simulink model "hw5_problem8"  (R2016a)
settings: Solver=VariableStepAuto  StartTime=-.005  StopTime=.5  RelTol=1e-3
values from neighbouring files (symbols this model uses):
  f_sw = 10e3    (= 10000)    [hw5.m]
  K_i_d = 10    [hw5.m]
  K_i_q = 10    [hw5.m]
  K_p_d = 100    [hw5.m]
  K_p_q = 100    [hw5.m]
  L = 3e-3    (= 0.003)    [hw5.m]
  R = .5    (= 0.5)    [hw5.m]
  theta_syn = w*t    (= 376.991118431)    [hw5.m]
  Vbus = 250    [hw5.m]
  w = 2*pi*60    (= 376.991118431)    [hw5.m]
libraries: dspsigops x4
settings Model: Creator=Seth Barger  LastModifiedBy=Seth Barger
settings DataIOCC: SaveOutput=off

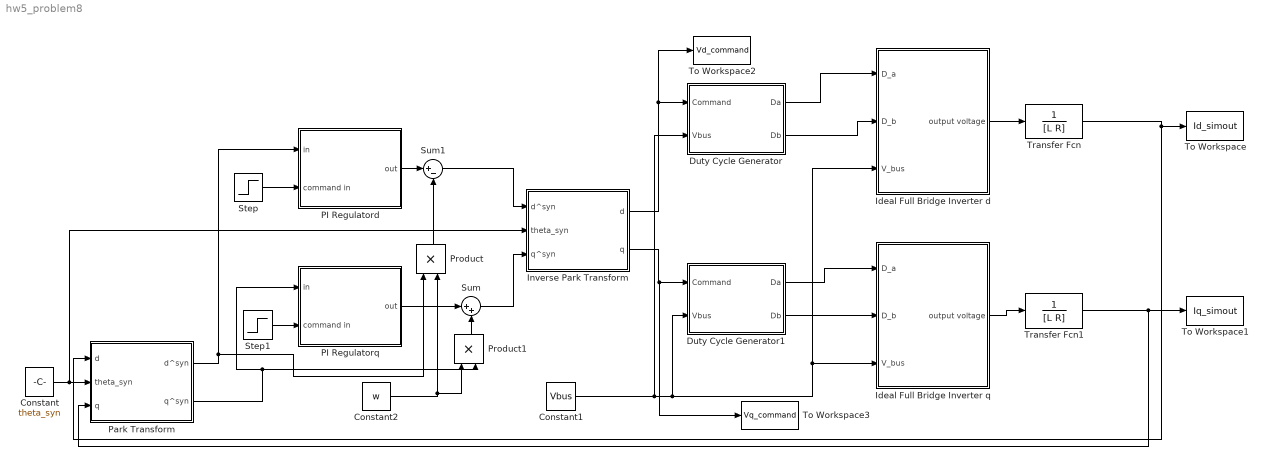
== system hw5_problem8 ==
  Constant : Constant  Value=theta_syn
  Constant1 : Constant  Value=Vbus
  Constant2 : Constant  Value=w
  Duty Cycle Generator : Subsystem
  Duty Cycle Generator1 : Subsystem
  "Ideal Full Bridge Inverter d " : Subsystem
  Ideal Full Bridge Inverter q : Subsystem
  Inverse Park Transform : Subsystem
  PI Regulatord : Subsystem
  PI Regulatorq : Subsystem
  Park Transform : Subsystem
  Product : Product
  Product1 : Product
  Step : Step  Time=0  After=20  SampleTime=0
  Step1 : Step  Time=0  After=-20  SampleTime=0
  Sum : Sum  Inputs=|++
  Sum1 : Sum  Inputs=|+-
  To Workspace : ToWorkspace  VariableName=Id_simout  SampleTime=-1
  To Workspace1 : ToWorkspace  VariableName=Iq_simout  SampleTime=-1
  To Workspace2 : ToWorkspace  VariableName=Vd_command  SampleTime=-1
  To Workspace3 : ToWorkspace  VariableName=Vq_command  SampleTime=-1
  Transfer Fcn : TransferFcn  Denominator=[L R]
  Transfer Fcn1 : TransferFcn  Denominator=[L R]
  wires:
  Constant/1 -> Inverse Park Transform/2(theta_syn), Park Transform/2(theta_syn)
  Park Transform/2(q^syn) -> Product1/2, PI Regulatorq/1(in)
  Park Transform/1(d^syn) -> Product/1, PI Regulatord/1(in)
  Constant1/1 -> Duty Cycle Generator/2(Vbus), Duty Cycle Generator1/2(Vbus), "Ideal Full Bridge Inverter d "/3(V_bus), Ideal Full Bridge Inverter q/3(V_bus)
  "Ideal Full Bridge Inverter d "/1(output voltage) -> Transfer Fcn/1
  Ideal Full Bridge Inverter q/1(output voltage) -> Transfer Fcn1/1
  Transfer Fcn1/1 -> To Workspace1/1, Park Transform/3(q)
  Transfer Fcn/1 -> To Workspace/1, Park Transform/1(d)
  Constant2/1 -> Product1/1, Product/2
  Product1/1 -> Sum/2
  PI Regulatorq/1(out) -> Sum/1
  Sum/1 -> Inverse Park Transform/3(q^syn)
  PI Regulatord/1(out) -> Sum1/1
  Product/1 -> Sum1/2
  Sum1/1 -> Inverse Park Transform/1(d^syn)
  Duty Cycle Generator/1(Da) -> "Ideal Full Bridge Inverter d "/1(D_a)
  Duty Cycle Generator/2(Db) -> "Ideal Full Bridge Inverter d "/2(D_b)
  Inverse Park Transform/1(d) -> To Workspace2/1, Duty Cycle Generator/1(Command)
  Duty Cycle Generator1/1(Da) -> Ideal Full Bridge Inverter q/1(D_a)
  Inverse Park Transform/2(q) -> To Workspace3/1, Duty Cycle Generator1/1(Command)
  Duty Cycle Generator1/2(Db) -> Ideal Full Bridge Inverter q/2(D_b)
  Step/1 -> PI Regulatord/2(command in)
  Step1/1 -> PI Regulatorq/2(command in)

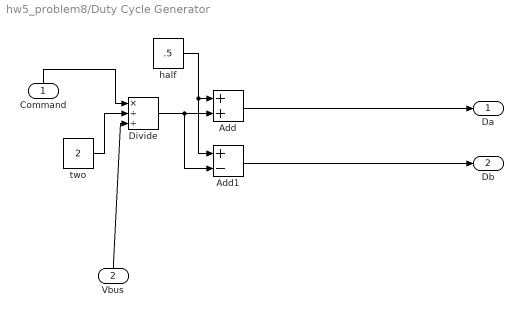
== system hw5_problem8/Duty Cycle Generator ==
  Command : Inport
  Vbus : Inport  Port=2
  Add : Sum
  Add1 : Sum  Inputs=+-
  Divide : Product  Inputs=*//
  half : Constant  Value=.5
  two : Constant  Value=2
  Da : Outport
  Db : Outport  Port=2
  wires:
  two/1 -> Divide/2
  Add/1 -> Da/1
  Command/1 -> Divide/1
  Vbus/1 -> Divide/3
  Divide/1 -> Add1/2, Add/2
  half/1 -> Add1/1, Add/1
  Add1/1 -> Db/1

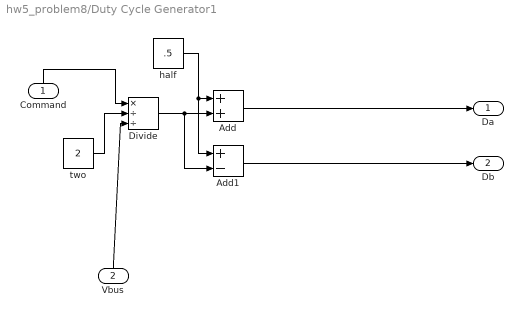
== system hw5_problem8/Duty Cycle Generator1 ==
  Command : Inport
  Vbus : Inport  Port=2
  Add : Sum
  Add1 : Sum  Inputs=+-
  Divide : Product  Inputs=*//
  half : Constant  Value=.5
  two : Constant  Value=2
  Da : Outport
  Db : Outport  Port=2
  wires:
  two/1 -> Divide/2
  Add/1 -> Da/1
  Command/1 -> Divide/1
  Vbus/1 -> Divide/3
  Divide/1 -> Add1/2, Add/2
  half/1 -> Add1/1, Add/1
  Add1/1 -> Db/1

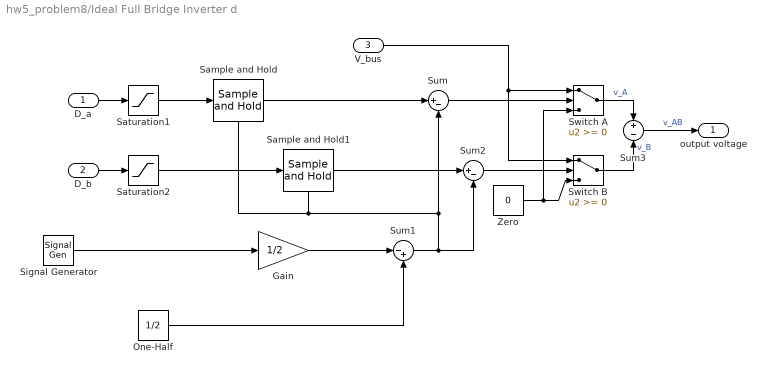
== system hw5_problem8/Ideal Full Bridge Inverter d  ==
  D_a : Inport
  D_b : Inport  Port=2
  V_bus : Inport  Port=3
  Gain : Gain  Gain=1/2  SaturateOnIntegerOverflow=on  OutDataTypeStr=Inherit: Same as input  ParamDataTypeStr=Inherit: Same as input
  One-Half : Constant  Value=1/2
  Sample and Hold : dspsigops/Sample and Hold  trig=Falling edge  initCond=0  latchinput=off
  Sample and Hold1 : dspsigops/Sample and Hold  trig=Falling edge  initCond=0  latchinput=off
  Saturation1 : Saturate  UpperLimit=1  LowerLimit=0
  Saturation2 : Saturate  UpperLimit=1  LowerLimit=0
  Signal Generator : SignalGenerator  WaveForm=sawtooth  Frequency=f_sw
  Sum : Sum  Inputs=|+-  SaturateOnIntegerOverflow=on
  Sum1 : Sum  Inputs=|-+  SaturateOnIntegerOverflow=on
  Sum2 : Sum  Inputs=|+-  SaturateOnIntegerOverflow=on
  Sum3 : Sum  Inputs=+-  SaturateOnIntegerOverflow=on
  Switch A : Switch  SaturateOnIntegerOverflow=on
  Switch B : Switch  SaturateOnIntegerOverflow=on
  Zero : Constant  Value=0
  output voltage : Outport
  wires:
  Sum/1 -> Switch A/2
  Zero/1 -> Switch A/3, Switch B/3
  Signal Generator/1 -> Gain/1
  Gain/1 -> Sum1/1
  One-Half/1 -> Sum1/2
  Sum2/1 -> Switch B/2
  Switch A/1 -> Sum3/1  "v_A"
  Switch B/1 -> Sum3/2  "v_B"
  Sum3/1 -> output voltage/1  "v_AB"
  Sum1/1 -> Sum2/2, Sample and Hold/Trigger, Sample and Hold1/Trigger, Sum/2
  V_bus/1 -> Switch A/1, Switch B/1
  D_a/1 -> Saturation1/1
  Sample and Hold/1 -> Sum/1
  D_b/1 -> Saturation2/1
  Sample and Hold1/1 -> Sum2/1
  Saturation1/1 -> Sample and Hold/1
  Saturation2/1 -> Sample and Hold1/1

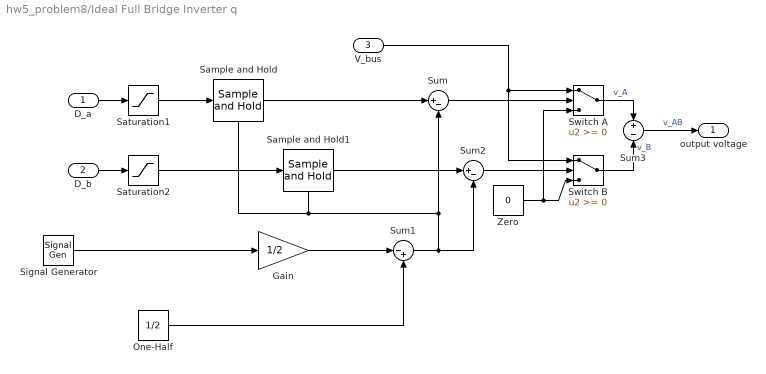
== system hw5_problem8/Ideal Full Bridge Inverter q ==
  D_a : Inport
  D_b : Inport  Port=2
  V_bus : Inport  Port=3
  Gain : Gain  Gain=1/2  SaturateOnIntegerOverflow=on  OutDataTypeStr=Inherit: Same as input  ParamDataTypeStr=Inherit: Same as input
  One-Half : Constant  Value=1/2
  Sample and Hold : dspsigops/Sample and Hold  trig=Falling edge  initCond=0  latchinput=off
  Sample and Hold1 : dspsigops/Sample and Hold  trig=Falling edge  initCond=0  latchinput=off
  Saturation1 : Saturate  UpperLimit=1  LowerLimit=0
  Saturation2 : Saturate  UpperLimit=1  LowerLimit=0
  Signal Generator : SignalGenerator  WaveForm=sawtooth  Frequency=f_sw
  Sum : Sum  Inputs=|+-  SaturateOnIntegerOverflow=on
  Sum1 : Sum  Inputs=|-+  SaturateOnIntegerOverflow=on
  Sum2 : Sum  Inputs=|+-  SaturateOnIntegerOverflow=on
  Sum3 : Sum  Inputs=+-  SaturateOnIntegerOverflow=on
  Switch A : Switch  SaturateOnIntegerOverflow=on
  Switch B : Switch  SaturateOnIntegerOverflow=on
  Zero : Constant  Value=0
  output voltage : Outport
  wires:
  Sum/1 -> Switch A/2
  Zero/1 -> Switch A/3, Switch B/3
  Signal Generator/1 -> Gain/1
  Gain/1 -> Sum1/1
  One-Half/1 -> Sum1/2
  Sum2/1 -> Switch B/2
  Switch A/1 -> Sum3/1  "v_A"
  Switch B/1 -> Sum3/2  "v_B"
  Sum3/1 -> output voltage/1  "v_AB"
  Sum1/1 -> Sum2/2, Sample and Hold/Trigger, Sample and Hold1/Trigger, Sum/2
  V_bus/1 -> Switch A/1, Switch B/1
  D_a/1 -> Saturation1/1
  Sample and Hold/1 -> Sum/1
  D_b/1 -> Saturation2/1
  Sample and Hold1/1 -> Sum2/1
  Saturation1/1 -> Sample and Hold/1
  Saturation2/1 -> Sample and Hold1/1

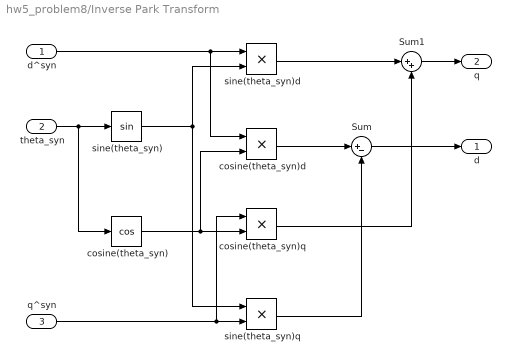
== system hw5_problem8/Inverse Park Transform ==
  d^syn : Inport
  theta_syn : Inport  Port=2
  q^syn : Inport  Port=3
  Sum : Sum  Inputs=|+-
  Sum1 : Sum  Inputs=|++
  cosine(theta_syn) : Trigonometry  Operator=cos
  cosine(theta_syn)d : Product
  cosine(theta_syn)q : Product
  sine(theta_syn) : Trigonometry
  sine(theta_syn)d : Product
  sine(theta_syn)q : Product
  d : Outport
  q : Outport  Port=2
  wires:
  Sum1/1 -> q/1
  cosine(theta_syn)q/1 -> Sum1/2
  cosine(theta_syn)d/1 -> Sum/1
  q^syn/1 -> cosine(theta_syn)q/1, sine(theta_syn)q/2
  sine(theta_syn)q/1 -> Sum/2
  cosine(theta_syn)/1 -> cosine(theta_syn)q/2, cosine(theta_syn)d/2
  Sum/1 -> d/1
  sine(theta_syn)d/1 -> Sum1/1
  theta_syn/1 -> cosine(theta_syn)/1, sine(theta_syn)/1
  d^syn/1 -> cosine(theta_syn)d/1, sine(theta_syn)d/1
  sine(theta_syn)/1 -> sine(theta_syn)q/1, sine(theta_syn)d/2

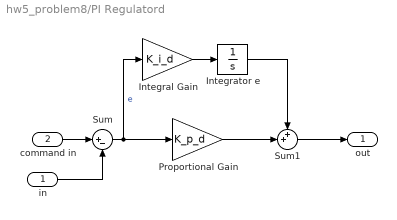
== system hw5_problem8/PI Regulatord ==
  in : Inport
  command in : Inport  Port=2
  Integral Gain : Gain  Gain=K_i_d  SaturateOnIntegerOverflow=on  OutDataTypeStr=Inherit: Same as input  ParamDataTypeStr=Inherit: Same as input
  Integrator e : Integrator
  Proportional Gain : Gain  Gain=K_p_d  SaturateOnIntegerOverflow=on  OutDataTypeStr=Inherit: Same as input  ParamDataTypeStr=Inherit: Same as input
  Sum : Sum  Inputs=|+-  SaturateOnIntegerOverflow=on
  Sum1 : Sum  Inputs=++|  SaturateOnIntegerOverflow=on
  out : Outport
  wires:
  Sum/1 -> Integral Gain/1, Proportional Gain/1  "e"
  command in/1 -> Sum/1
  in/1 -> Sum/2
  Proportional Gain/1 -> Sum1/2
  Sum1/1 -> out/1
  Integral Gain/1 -> Integrator e/1
  Integrator e/1 -> Sum1/1

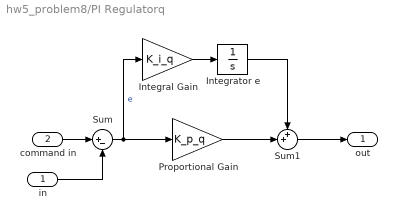
== system hw5_problem8/PI Regulatorq ==
  in : Inport
  command in : Inport  Port=2
  Integral Gain : Gain  Gain=K_i_q  SaturateOnIntegerOverflow=on  OutDataTypeStr=Inherit: Same as input  ParamDataTypeStr=Inherit: Same as input
  Integrator e : Integrator
  Proportional Gain : Gain  Gain=K_p_q  SaturateOnIntegerOverflow=on  OutDataTypeStr=Inherit: Same as input  ParamDataTypeStr=Inherit: Same as input
  Sum : Sum  Inputs=|+-  SaturateOnIntegerOverflow=on
  Sum1 : Sum  Inputs=++|  SaturateOnIntegerOverflow=on
  out : Outport
  wires:
  Sum/1 -> Integral Gain/1, Proportional Gain/1  "e"
  command in/1 -> Sum/1
  in/1 -> Sum/2
  Proportional Gain/1 -> Sum1/2
  Sum1/1 -> out/1
  Integral Gain/1 -> Integrator e/1
  Integrator e/1 -> Sum1/1

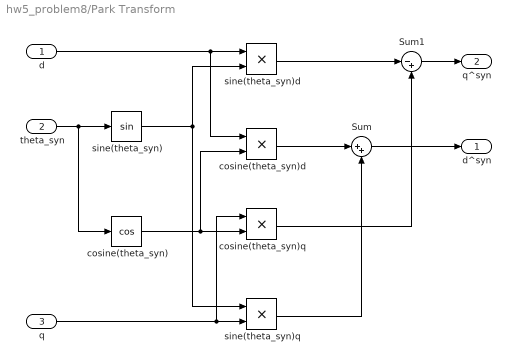
== system hw5_problem8/Park Transform ==
  d : Inport
  theta_syn : Inport  Port=2
  q : Inport  Port=3
  Sum : Sum  Inputs=|++
  Sum1 : Sum  Inputs=|-+
  cosine(theta_syn) : Trigonometry  Operator=cos
  cosine(theta_syn)d : Product
  cosine(theta_syn)q : Product
  sine(theta_syn) : Trigonometry
  sine(theta_syn)d : Product
  sine(theta_syn)q : Product
  d^syn : Outport
  q^syn : Outport  Port=2
  wires:
  Sum1/1 -> q^syn/1
  cosine(theta_syn)q/1 -> Sum1/2
  cosine(theta_syn)d/1 -> Sum/1
  q/1 -> cosine(theta_syn)q/1, sine(theta_syn)q/2
  sine(theta_syn)q/1 -> Sum/2
  cosine(theta_syn)/1 -> cosine(theta_syn)q/2, cosine(theta_syn)d/2
  Sum/1 -> d^syn/1
  sine(theta_syn)d/1 -> Sum1/1
  theta_syn/1 -> cosine(theta_syn)/1, sine(theta_syn)/1
  d/1 -> cosine(theta_syn)d/1, sine(theta_syn)d/1
  sine(theta_syn)/1 -> sine(theta_syn)q/1, sine(theta_syn)d/2
